simulink model "Aula_Simulink"  (R2019a)
settings: Solver=VariableStepAuto  StartTime=0.0  StopTime=30  RelTol=1e-3
settings Model: Creator=vinic  LastModifiedBy=vinic
settings DataIOCC: ReturnWorkspaceOutputs=off
settings DebuggingCC: PregeneratedLibrarySubsystemCodeDiagnostic=none  ArithmeticOperatorsInVariantConditions=warning
settings SFSimCC: SimUseLocalCustomCode=off
settings RTWCC: RTWUseLocalCustomCode=off

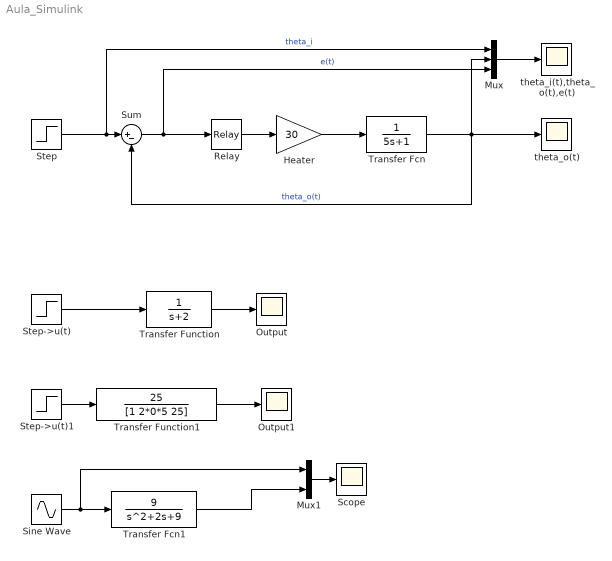
== system Aula_Simulink ==
  Heater : Gain  Gain=30
  Mux : Mux  Inputs=3
  Mux1 : Mux  Inputs=2
  Output : Scope
  Output1 : Scope
  Relay : Relay  OnSwitchValue=2  OffSwitchValue=-2
  Scope : Scope
  Sine Wave : Sin  SampleTime=0
  Step : Step  Time=0  After=22  SampleTime=0
  Step->u(t) : Step  Time=0  After=10  SampleTime=0
  Step->u(t)1 : Step  Time=0  After=10  SampleTime=0
  Sum : Sum  Inputs=|+-
  Transfer Fcn : TransferFcn  Denominator=[5 1]
  Transfer Fcn1 : TransferFcn  Numerator=[9]  Denominator=[1 2 9]
  Transfer Function : TransferFcn  Denominator=[1 2]
  Transfer Function1 : TransferFcn  Numerator=[25]  Denominator=[1 2*0*5 25]
  theta_i(t),theta_o(t),e(t) : Scope
  theta_o(t) : Scope
  wires:
  Transfer Fcn/1 -> theta_o(t)/1, Sum/2, Mux/2  "theta_o(t)"
  Mux/1 -> theta_i(t),theta_o(t),e(t)/1
  Step/1 -> Sum/1, Mux/1  "theta_i"
  Relay/1 -> Heater/1
  Sum/1 -> Mux/3, Relay/1  "e(t)"
  Heater/1 -> Transfer Fcn/1
  Step->u(t)/1 -> Transfer Function/1
  Transfer Function/1 -> Output/1
  Transfer Function1/1 -> Output1/1
  Step->u(t)1/1 -> Transfer Function1/1
  Sine Wave/1 -> Mux1/1, Transfer Fcn1/1
  Mux1/1 -> Scope/1
  Transfer Fcn1/1 -> Mux1/2
